simulink model "Top_Level_Model"  (R2023a)
settings: Solver=VariableStepAuto  StartTime=0.0  StopTime=10.0  RelTol=1e-3
settings Model: Creator=hunte  LastModifiedBy=hunte

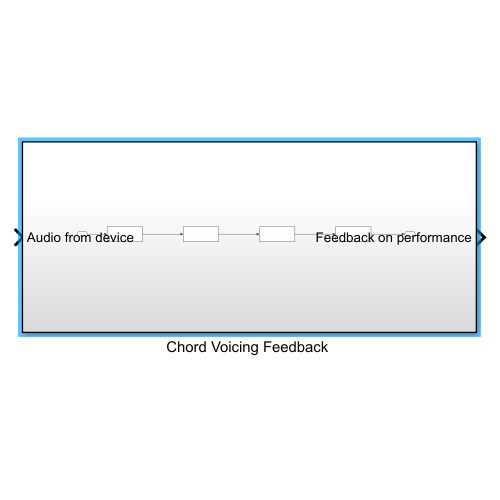
[thumbnail: Simulink's stored preview of the top-level diagram]
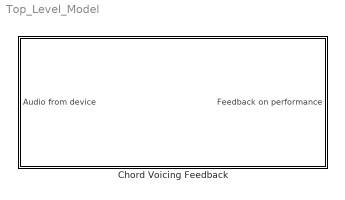
== system Top_Level_Model ==
  "Chord Voicing Feedback " : Subsystem

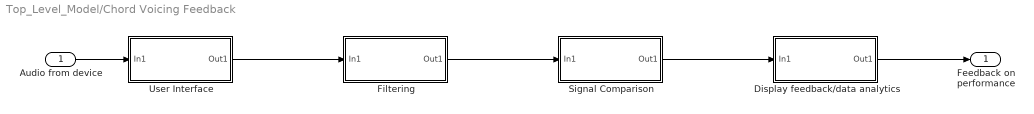
== system Top_Level_Model/Chord Voicing Feedback  ==
  Audio from device : Inport
  Display feedback/data analytics : Subsystem
  Filtering : Subsystem
  Signal Comparison : Subsystem
  User Interface : Subsystem
  Feedback on performance : Outport
  wires:
  User Interface/1(Out1) -> Filtering/1(In1)
  Display feedback/data analytics/1(Out1) -> Feedback on performance/1
  Audio from device/1 -> User Interface/1(In1)
  Filtering/1(Out1) -> Signal Comparison/1(In1)
  Signal Comparison/1(Out1) -> Display feedback/data analytics/1(In1)

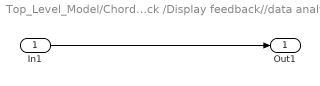
== system Top_Level_Model/Chord Voicing Feedback /Display feedback//data analytics ==
  In1 : Inport
  Out1 : Outport
  wires:
  In1/1 -> Out1/1

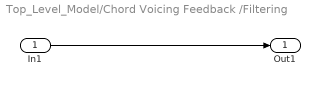
== system Top_Level_Model/Chord Voicing Feedback /Filtering ==
  In1 : Inport
  Out1 : Outport
  wires:
  In1/1 -> Out1/1

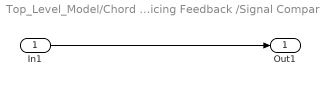
== system Top_Level_Model/Chord Voicing Feedback /Signal Comparison ==
  In1 : Inport
  Out1 : Outport
  wires:
  In1/1 -> Out1/1

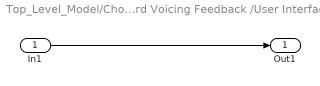
== system Top_Level_Model/Chord Voicing Feedback /User Interface ==
  In1 : Inport
  Out1 : Outport
  wires:
  In1/1 -> Out1/1
